simulink model "Modelo_NL_CONTROL_INTERNO_VECTORIAL"  (R2017a)
settings: Solver=VariableStepAuto  StartTime=0.0  StopTime=1  MaxStep=1e-4  RelTol=1e-3
values from neighbouring files (symbols this model uses):
  alfa_cu = 3.9e-3    (= 0.0039)    [modelo_global_NL.m]
  beq = bl/r^2 + bm    (= 1.5638971155e-05)    [Evaluacion_polos_5_2_2.m]    (also in modelo_global_NL.m = 1.5e-05)
  Cts = 0.818    [modelo_global_NL.m]
  Jeq = Jl/r^2 + Jm    (= 6.9338269301e-06)    [Evaluacion_polos_5_2_2.m]    (also in modelo_global_NL.m = 5.65588462007e-06)
  LambdaM = 0.01546    [Evaluacion_polos_5_2_2.m]    (also in modelo_global_NL.m)
  Ld = 0.0066    [Evaluacion_polos_5_2_2.m]    (also in modelo_global_NL.m)
  Lq = 0.0058    [Evaluacion_polos_5_2_2.m]    (also in modelo_global_NL.m)
  Pp = 3    [Evaluacion_polos_5_2_2.m]    (also in modelo_global_NL.m)
  R0 = 4    [Evaluacion_polos_5_2_2.m]    (also in modelo_global_NL.m)
  Rd = 33    [Evaluacion_polos_5_2_2.m]    (also in modelo_global_NL.m)
  Rq = 29    [Evaluacion_polos_5_2_2.m]    (also in modelo_global_NL.m)
  Rsref = 1.02    [modelo_global_NL.m]
  Rts_amb = 146.7    [modelo_global_NL.m]
  Tamb = 40    [modelo_global_NL.m]
  Tsref = 40    [modelo_global_NL.m]
undefined symbols (not defined in the file or in its folder): sigbuilder_block
settings Model: Creator=merem  LastModifiedBy=merem

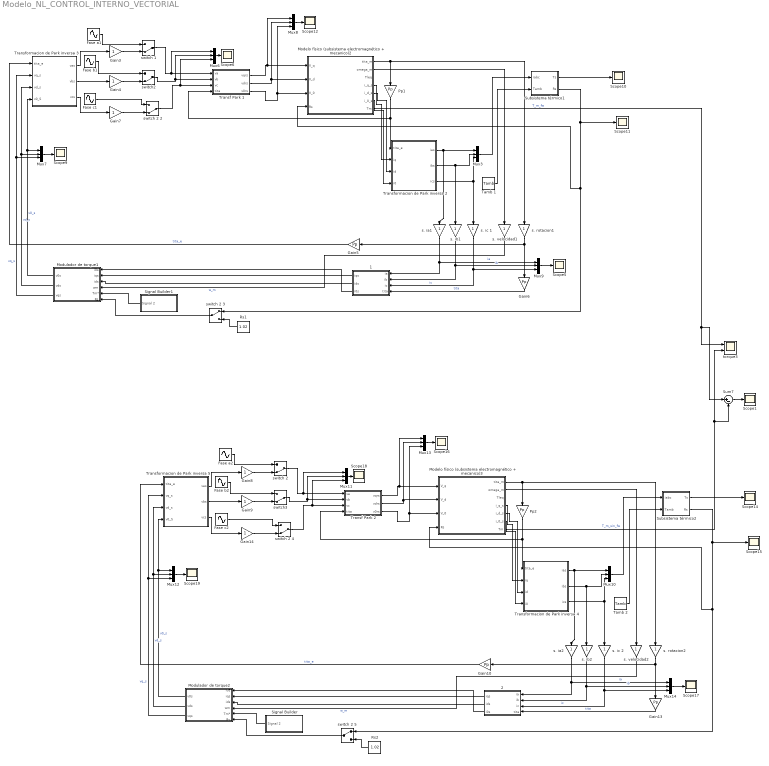
== system Modelo_NL_CONTROL_INTERNO_VECTORIAL ==
  " 1" : Subsystem
  " 2" : Subsystem
  Fase a1 : Sin  SampleTime=0
  Fase a2 : Sin  SampleTime=0
  Fase b1 : Sin  SampleTime=0
  Fase b2 : Sin  SampleTime=0
  Fase c1 : Sin  SampleTime=0
  Fase c2 : Sin  SampleTime=0
  Gain{5..6,10,13} (4 alike) : Gain  Gain=Pp
  Gain{3..4,7..9,14} (6 alike) : Gain
  Modelo físico (subsistema electromagnético + mecanico)2 : Subsystem
  Modelo físico (subsistema electromagnético + mecanico)3 : Subsystem
  Modulador de torque1 : Subsystem
  Modulador de torque2 : Subsystem
  Mux{3,6..14} (10 alike) : Mux  Inputs=3
  Pp1 : Gain  Gain=Pp
  Pp2 : Gain  Gain=Pp
  Rs1 : Constant  Value=1.02
  Rs2 : Constant  Value=1.02
  Scope{1,5..6,9..12,14..19} (13 alike) : Scope
  Signal Builder : Subsystem  Tag=STV Subsys  LoadFcn=sigbuilder_block('load');  StartFcn=sigbuilder_block('start');  StopFcn=sigbuilder_block('stop');  ClipboardFcn=sigbuilder_block('clipboard');  mask(Sigbuilder block){tuvar=[0:10]}
      mask help: Simulink:masks:SigbuilderBlock_MD
      mask init:
      | if ~strcmp(get_param(bdroot(gcbh),'SimulationStatus'),'stopped') tuvar = sigbuilder_block('maskInit'); end
      settings: CopyFcn=sigbuilder_block('copy');  DeleteFcn=sigbuilder_block('delete');  ModelCloseFcn=sigbuilder_block('modelClose');  PreSaveFcn=sigbuilder_block('preSave');  PauseFcn=sigbuilder_block('pause');  ContinueFcn=sigbuilder_block('continue');  NameChangeFcn=sigbuilder_block('namechange');  OpenFcn=sigbuilder_block('open',[6 30 1012.5 447.75 ]);  CloseFcn=sigbuilder_block('close');
      mask Display: plot(0, 0, 100, 100,[2, 2, 32, 32, 2], [68, 8, 8, 68, 68],[32, 2], [38, 38], [32, 19, 2],[53, 60, 44], [32, 17, 17, 2],[16, 16, 31, 31]);txt = getActiveGroup(gcbh);text(2, 100, txt,'verticalAlignment', 'top');
  Signal Builder1 : Subsystem  Tag=STV Subsys  LoadFcn=sigbuilder_block('load');  StartFcn=sigbuilder_block('start');  StopFcn=sigbuilder_block('stop');  ClipboardFcn=sigbuilder_block('clipboard');  mask(Sigbuilder block){tuvar=[0:10]}
      mask help: Simulink:masks:SigbuilderBlock_MD
      mask init:
      | if ~strcmp(get_param(bdroot(gcbh),'SimulationStatus'),'stopped') tuvar = sigbuilder_block('maskInit'); end
      settings: CopyFcn=sigbuilder_block('copy');  DeleteFcn=sigbuilder_block('delete');  ModelCloseFcn=sigbuilder_block('modelClose');  PreSaveFcn=sigbuilder_block('preSave');  PauseFcn=sigbuilder_block('pause');  ContinueFcn=sigbuilder_block('continue');  NameChangeFcn=sigbuilder_block('namechange');  OpenFcn=sigbuilder_block('open',[6 30 1012.5 447.75 ]);  CloseFcn=sigbuilder_block('close');
      mask Display: plot(0, 0, 100, 100,[2, 2, 32, 32, 2], [68, 8, 8, 68, 68],[32, 2], [38, 38], [32, 19, 2],[53, 60, 44], [32, 17, 17, 2],[16, 16, 31, 31]);txt = getActiveGroup(gcbh);text(2, 100, txt,'verticalAlignment', 'top');
  Subsistema térmico1 : Subsystem
  Subsistema térmico2 : Subsystem
  Sum7 : Sum  Inputs=|+-
  Tamb 1 : Constant  Value=Tamb
  Tamb 2 : Constant  Value=Tamb
  Transf Park 1 : Subsystem
  Transf Park 2 : Subsystem
  Transformacion de Park inversa 2 : Subsystem
  Transformacion de Park inversa 3 : Subsystem
  Transformacion de Park inversa 4 : Subsystem
  Transformacion de Park inversa 5 : Subsystem
  s. ia1 : Gain
  s. ia2 : Gain
  s. ib1 : Gain
  s. ib2 : Gain
  s. ic 1 : Gain
  s. ic 2 : Gain
  s. rotacion1 : Gain
  s. rotacion2 : Gain
  s. velocidad1 : Gain
  s. velocidad2 : Gain
  switch 1 : ManualSwitch  CurrentSetting=0
  switch 2 : ManualSwitch  CurrentSetting=0
  switch 2 2 : ManualSwitch  CurrentSetting=0
  switch 2 3 : ManualSwitch
  switch 2 4 : ManualSwitch  CurrentSetting=0
  switch 2 5 : ManualSwitch
  switch2 : ManualSwitch  CurrentSetting=0
  switch3 : ManualSwitch  CurrentSetting=0
  torque3 : Scope  NumInputPorts=2
  wires:
  Gain3/1 -> switch 1/2
  Modulador de torque1/2(vds) -> Mux7/2, Transformacion de Park inversa 3/3(vd_s)  "vd_s"
  " 1"/1(iqs) -> Modulador de torque1/2(iqs)
  Mux9/1 -> Scope5/1
  Gain6/1 -> " 1"/4("tita ")  "tita"
  s. rotacion1/1 -> Gain6/1, Gain5/1
  switch 2 2/1 -> Mux6/3, Transf Park 1/3(vc)
  Gain7/1 -> switch 2 2/2
  s. ib1/1 -> Mux9/2, " 1"/2("ib ")  "ib"
  Transformacion de Park inversa 2/3("ics ") -> Mux3/3, s. ic 1/1
  Gain4/1 -> switch2/2
  Fase c1/1 -> switch 2 2/1
  Subsistema térmico1/1(Ts) -> Scope10/1
  Transformacion de Park inversa 3/2(vbs) -> Gain4/1
  s. velocidad1/1 -> Modulador de torque1/4(wm)  "w_m"
  switch2/1 -> Mux6/2, Transf Park 1/2(vb)
  Modelo físico (subsistema electromagnético + mecanico)2/4("i_q_s ") -> Transformacion de Park inversa 2/2(iq)
  s. ia1/1 -> Mux9/1, " 1"/1("ia ")  "ia"
  Transf Park 1/2("vdrs ") -> Modelo físico (subsistema electromagnético + mecanico)2/2(V_d), Mux8/2
  Transformacion de Park inversa 2/1(ias) -> Mux3/1, s. ia1/1
  " 1"/2("ids ") -> Modulador de torque1/3(ids)
  Fase a1/1 -> switch 1/1
  s. ic 1/1 -> Mux9/3, " 1"/3("ic ")  "ic"
  switch 2 3/1 -> Modulador de torque1/6(Rs)
  Mux3/1 -> Subsistema térmico1/1(iabc)
  Transformacion de Park inversa 3/3("vcs ") -> Gain7/1
  Tamb 1/1 -> Subsistema térmico1/2("Tamb ")
  Modulador de torque1/3(vqs) -> Mux7/3, Transformacion de Park inversa 3/2(vq_s)  "vq_s"
  Mux7/1 -> Scope9/1
  Rs1/1 -> switch 2 3/2
  Pp1/1 -> Transf Park 1/4(tita), Transformacion de Park inversa 2/1(tita_e)
  " 1"/3("i0s ") -> Modulador de torque1/1(i0s)
  Transf Park 1/3("v0rs ") -> Modelo físico (subsistema electromagnético + mecanico)2/3(V_0), Mux8/3
  Transformacion de Park inversa 3/1(vas) -> Gain3/1
  Transf Park 1/1(vqrs) -> Modelo físico (subsistema electromagnético + mecanico)2/1(V_q), Mux8/1
  Fase b1/1 -> switch2/1
  switch 1/1 -> Mux6/1, Transf Park 1/1("va ")
  Mux8/1 -> Scope12/1
  Modelo físico (subsistema electromagnético + mecanico)2/6("i_0_s ") -> Transformacion de Park inversa 2/4(i0)
  Modelo físico (subsistema electromagnético + mecanico)2/5("i_d_s ") -> Transformacion de Park inversa 2/3(id)
  Transformacion de Park inversa 2/2(ibs) -> Mux3/2, s. ib1/1
  Modelo físico (subsistema electromagnético + mecanico)2/1("tita_m ") -> Pp1/1, s. rotacion1/1
  Subsistema térmico1/2("Rs ") -> Scope11/1, Modelo físico (subsistema electromagnético + mecanico)2/4(Rs), switch 2 3/1
  Modulador de torque1/1(v0s) -> Mux7/1, Transformacion de Park inversa 3/4("v0_S ")  "v0_s"
  Gain5/1 -> Transformacion de Park inversa 3/1(tita_e)  "tita_e"
  Mux6/1 -> Scope6/1
  Gain8/1 -> switch 2/2
  " 2"/1(iqs) -> Modulador de torque2/2(iqs)
  Modulador de torque2/2(vds) -> Mux12/2, Transformacion de Park inversa 5/3(vd_s)  "vd_s"
  Gain9/1 -> switch3/2
  s. velocidad2/1 -> Modulador de torque2/4(wm)  "w_m"
  Subsistema térmico2/1(Ts) -> Scope14/1
  s. ib2/1 -> Mux14/2, " 2"/2("ib ")  "ib"
  Gain14/1 -> switch 2 4/2
  Gain13/1 -> " 2"/4("tita ")  "tita"
  Transformacion de Park inversa 5/1(vas) -> Gain8/1
  Mux14/1 -> Scope17/1
  Gain10/1 -> Transformacion de Park inversa 5/1(tita_e)  "tita_e"
  Transformacion de Park inversa 4/2(ibs) -> Mux10/2, s. ib2/1
  Mux11/1 -> Scope18/1
  Modulador de torque2/1(v0s) -> Mux12/1, Transformacion de Park inversa 5/4("v0_S ")  "v0_s"
  Modelo físico (subsistema electromagnético + mecanico)3/5("i_d_s ") -> Transformacion de Park inversa 4/3(id)
  switch 2 4/1 -> Mux11/3, Transf Park 2/3(vc)
  Pp2/1 -> Transf Park 2/4(tita), Transformacion de Park inversa 4/1(tita_e)
  Transf Park 2/2("vdrs ") -> Modelo físico (subsistema electromagnético + mecanico)3/2(V_d), Mux13/2
  s. rotacion2/1 -> Gain13/1, Gain10/1
  Transformacion de Park inversa 5/3("vcs ") -> Gain14/1
  Modulador de torque2/3(vqs) -> Mux12/3, Transformacion de Park inversa 5/2(vq_s)  "vq_s"
  " 2"/2("ids ") -> Modulador de torque2/3(ids)
  Transformacion de Park inversa 5/2(vbs) -> Gain9/1
  s. ia2/1 -> Mux14/1, " 2"/1("ia ")  "ia"
  switch3/1 -> Mux11/2, Transf Park 2/2(vb)
  Modelo físico (subsistema electromagnético + mecanico)3/4("i_q_s ") -> Transformacion de Park inversa 4/2(iq)
  switch 2 5/1 -> Modulador de torque2/6(Rs)
  Fase c2/1 -> switch 2 4/1
  Modelo físico (subsistema electromagnético + mecanico)3/1("tita_m ") -> Pp2/1, s. rotacion2/1
  Transformacion de Park inversa 4/1(ias) -> Mux10/1, s. ia2/1
  Mux10/1 -> Subsistema térmico2/1(iabc)
  switch 2/1 -> Mux11/1, Transf Park 2/1("va ")
  Tamb 2/1 -> Subsistema térmico2/2("Tamb ")
  Transf Park 2/1(vqrs) -> Modelo físico (subsistema electromagnético + mecanico)3/1(V_q), Mux13/1
  Modelo físico (subsistema electromagnético + mecanico)3/6("i_0_s ") -> Transformacion de Park inversa 4/4(i0)
  Transformacion de Park inversa 4/3("ics ") -> Mux10/3, s. ic 2/1
  Mux12/1 -> Scope19/1
  " 2"/3("i0s ") -> Modulador de torque2/1(i0s)
  Mux13/1 -> Scope16/1
  Fase a2/1 -> switch 2/1
  s. ic 2/1 -> Mux14/3, " 2"/3("ic ")  "ic"
  Transf Park 2/3("v0rs ") -> Modelo físico (subsistema electromagnético + mecanico)3/3(V_0), Mux13/3
  Fase b2/1 -> switch3/1
  Rs2/1 -> switch 2 5/2
  Subsistema térmico2/2("Rs ") -> Scope15/1, Modelo físico (subsistema electromagnético + mecanico)3/4(Rs), switch 2 5/1
  Modelo físico (subsistema electromagnético + mecanico)3/7(Tm) -> Sum7/2, torque3/2  "T_m_sin_fw"
  Modelo físico (subsistema electromagnético + mecanico)2/7(Tm) -> Sum7/1, torque3/1  "T_m_fw"
  Signal Builder/1(Signal 2) -> Modulador de torque2/5(Tm*)
  Signal Builder1/1(Signal 2) -> Modulador de torque1/5(Tm*)
  Modelo físico (subsistema electromagnético + mecanico)2/2("omega_m ") -> s. velocidad1/1
  Modelo físico (subsistema electromagnético + mecanico)3/2("omega_m ") -> s. velocidad2/1
  Sum7/1 -> Scope1/1

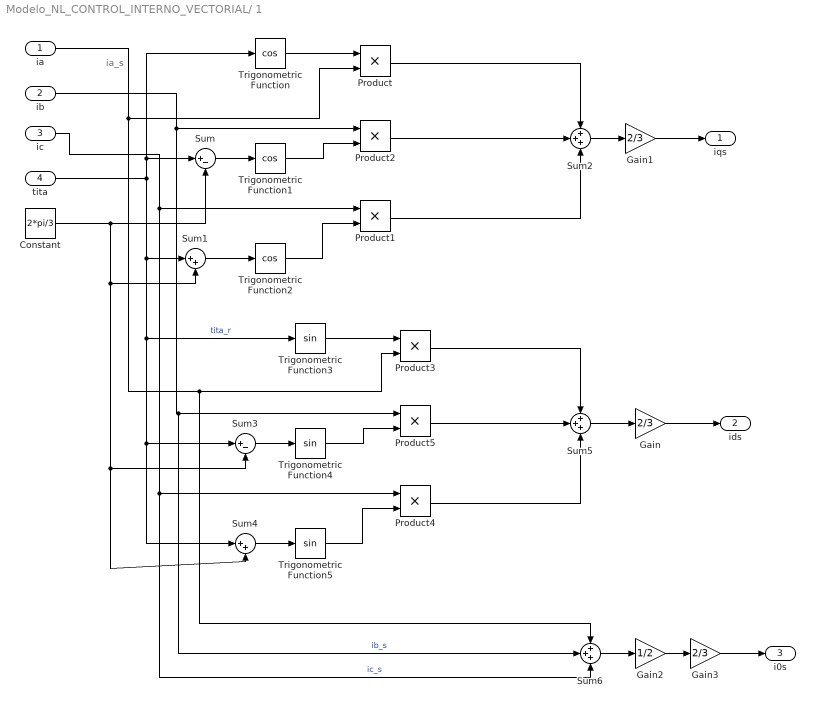
== system Modelo_NL_CONTROL_INTERNO_VECTORIAL/ 1 ==
  note: ia_s
  "ia " : Inport
  "ib " : Inport  Port=2
  "ic " : Inport  Port=3
  "tita " : Inport  Port=4
  Constant : Constant  Value=2*pi/3
  Gain : Gain  Gain=2/3
  Gain1 : Gain  Gain=2/3
  Gain2 : Gain  Gain=1/2
  Gain3 : Gain  Gain=2/3
  Product{,1..5} (6 alike) : Product
  Sum : Sum  Inputs=|+-
  Sum1 : Sum  Inputs=|++
  Sum2 : Sum  Inputs=+++
  Sum3 : Sum  Inputs=|+-
  Sum4 : Sum  Inputs=|++
  Sum5 : Sum  Inputs=+++
  Sum6 : Sum  Inputs=+++
  Trigonometric Function : Trigonometry  Operator=cos
  Trigonometric Function1 : Trigonometry  Operator=cos
  Trigonometric Function2 : Trigonometry  Operator=cos
  Trigonometric Function3 : Trigonometry
  Trigonometric Function4 : Trigonometry
  Trigonometric Function5 : Trigonometry
  iqs : Outport
  "ids " : Outport  Port=2
  "i0s " : Outport  Port=3
  wires:
  "tita "/1 -> Trigonometric Function/1, Sum/1, Sum1/1, Trigonometric Function3/1, Sum3/1, Sum4/1  "tita_r"
  Trigonometric Function/1 -> Product/1
  "ia "/1 -> Sum6/1, Product3/2, Product/2
  Constant/1 -> Sum4/2, Sum3/2, Sum1/2, Sum/2
  Sum/1 -> Trigonometric Function1/1
  Sum1/1 -> Trigonometric Function2/1
  Trigonometric Function1/1 -> Product2/2
  Trigonometric Function2/1 -> Product1/2
  "ib "/1 -> Sum6/2, Product5/1, Product2/1  "ib_s"
  "ic "/1 -> Sum6/3, Product4/1, Product1/1  "ic_s"
  Product/1 -> Sum2/1
  Product2/1 -> Sum2/2
  Sum2/1 -> Gain1/1
  Trigonometric Function5/1 -> Product4/2
  Trigonometric Function3/1 -> Product3/1
  Sum4/1 -> Trigonometric Function5/1
  Sum3/1 -> Trigonometric Function4/1
  Trigonometric Function4/1 -> Product5/2
  Product3/1 -> Sum5/1
  Product5/1 -> Sum5/2
  Product4/1 -> Sum5/3
  Sum5/1 -> Gain/1
  Product1/1 -> Sum2/3
  Gain/1 -> "ids "/1
  Gain1/1 -> iqs/1
  Sum6/1 -> Gain2/1
  Gain2/1 -> Gain3/1
  Gain3/1 -> "i0s "/1

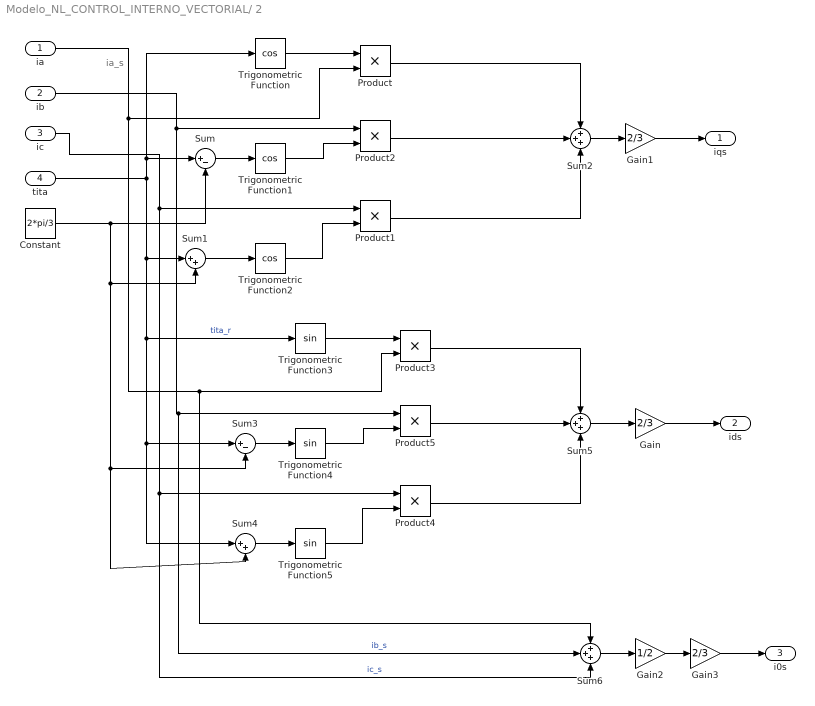
== system Modelo_NL_CONTROL_INTERNO_VECTORIAL/ 2 ==
  note: ia_s
  "ia " : Inport
  "ib " : Inport  Port=2
  "ic " : Inport  Port=3
  "tita " : Inport  Port=4
  Constant : Constant  Value=2*pi/3
  Gain : Gain  Gain=2/3
  Gain1 : Gain  Gain=2/3
  Gain2 : Gain  Gain=1/2
  Gain3 : Gain  Gain=2/3
  Product{,1..5} (6 alike) : Product
  Sum : Sum  Inputs=|+-
  Sum1 : Sum  Inputs=|++
  Sum2 : Sum  Inputs=+++
  Sum3 : Sum  Inputs=|+-
  Sum4 : Sum  Inputs=|++
  Sum5 : Sum  Inputs=+++
  Sum6 : Sum  Inputs=+++
  Trigonometric Function : Trigonometry  Operator=cos
  Trigonometric Function1 : Trigonometry  Operator=cos
  Trigonometric Function2 : Trigonometry  Operator=cos
  Trigonometric Function3 : Trigonometry
  Trigonometric Function4 : Trigonometry
  Trigonometric Function5 : Trigonometry
  iqs : Outport
  "ids " : Outport  Port=2
  "i0s " : Outport  Port=3
  wires:
  "tita "/1 -> Trigonometric Function/1, Sum/1, Sum1/1, Trigonometric Function3/1, Sum3/1, Sum4/1  "tita_r"
  Trigonometric Function/1 -> Product/1
  "ia "/1 -> Sum6/1, Product3/2, Product/2
  Constant/1 -> Sum4/2, Sum3/2, Sum1/2, Sum/2
  Sum/1 -> Trigonometric Function1/1
  Sum1/1 -> Trigonometric Function2/1
  Trigonometric Function1/1 -> Product2/2
  Trigonometric Function2/1 -> Product1/2
  "ib "/1 -> Sum6/2, Product5/1, Product2/1  "ib_s"
  "ic "/1 -> Sum6/3, Product4/1, Product1/1  "ic_s"
  Product/1 -> Sum2/1
  Product2/1 -> Sum2/2
  Sum2/1 -> Gain1/1
  Trigonometric Function5/1 -> Product4/2
  Trigonometric Function3/1 -> Product3/1
  Sum4/1 -> Trigonometric Function5/1
  Sum3/1 -> Trigonometric Function4/1
  Trigonometric Function4/1 -> Product5/2
  Product3/1 -> Sum5/1
  Product5/1 -> Sum5/2
  Product4/1 -> Sum5/3
  Sum5/1 -> Gain/1
  Product1/1 -> Sum2/3
  Gain/1 -> "ids "/1
  Gain1/1 -> iqs/1
  Sum6/1 -> Gain2/1
  Gain2/1 -> Gain3/1
  Gain3/1 -> "i0s "/1

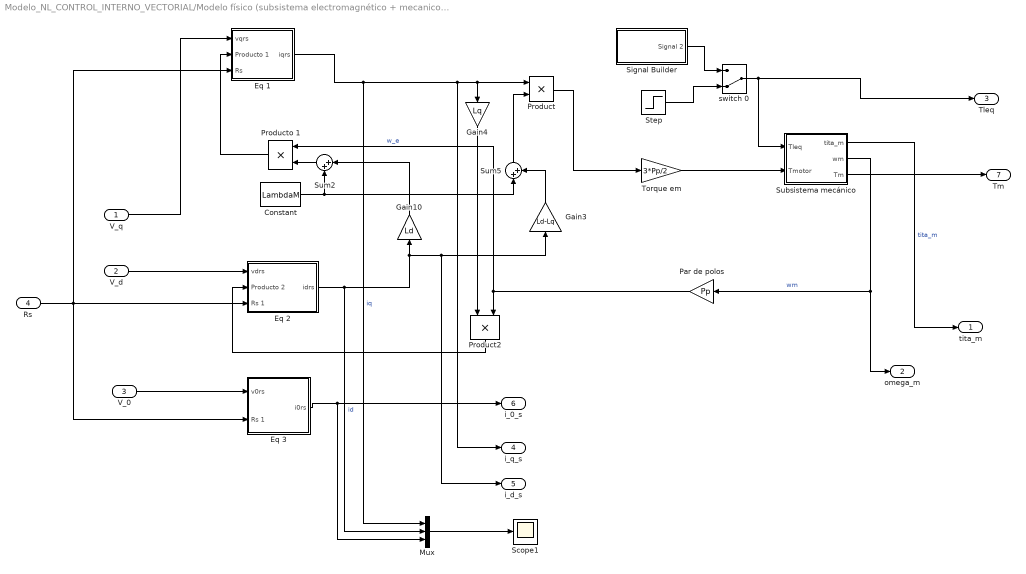
== system Modelo_NL_CONTROL_INTERNO_VECTORIAL/Modelo físico (subsistema electromagnético + mecanico)2 ==
  V_q : Inport
  V_d : Inport  Port=2
  V_0 : Inport  Port=3
  Rs : Inport  Port=4
  Constant : Constant  Value=LambdaM
  Eq 1 : Subsystem
  "Eq 2 " : Subsystem
  Eq 3 : Subsystem
  Gain10 : Gain  Gain=Ld
  Gain3 : Gain  Gain=Ld-Lq
  Gain4 : Gain  Gain=Lq
  Mux : Mux  Inputs=3
  Par de polos : Gain  Gain=Pp
  Product : Product
  Product2 : Product
  Producto 1 : Product
  Scope1 : Scope
  Signal Builder : Subsystem  Tag=STV Subsys  LoadFcn=sigbuilder_block('load');  StartFcn=sigbuilder_block('start');  StopFcn=sigbuilder_block('stop');  ClipboardFcn=sigbuilder_block('clipboard');  mask(Sigbuilder block){tuvar=[0:10]}
      mask help: Simulink:masks:SigbuilderBlock_MD
      mask init:
      | if ~strcmp(get_param(bdroot(gcbh),'SimulationStatus'),'stopped') tuvar = sigbuilder_block('maskInit'); end
      settings: CopyFcn=sigbuilder_block('copy');  DeleteFcn=sigbuilder_block('delete');  ModelCloseFcn=sigbuilder_block('modelClose');  PreSaveFcn=sigbuilder_block('preSave');  PauseFcn=sigbuilder_block('pause');  ContinueFcn=sigbuilder_block('continue');  NameChangeFcn=sigbuilder_block('namechange');  OpenFcn=sigbuilder_block('open',[6 30 1012.5 447.75 ]);  CloseFcn=sigbuilder_block('close');
      mask Display: plot(0, 0, 100, 100,[2, 2, 32, 32, 2], [68, 8, 8, 68, 68],[32, 2], [38, 38], [32, 19, 2],[53, 60, 44], [32, 17, 17, 2],[16, 16, 31, 31]);txt = getActiveGroup(gcbh);text(2, 100, txt,'verticalAlignment', 'top');
  Step : Step  Time=0.3  After=0  SampleTime=0
  Subsistema mecánico : Subsystem
  Sum2 : Sum  Inputs=|++
  Sum5 : Sum  Inputs=|++
  "Torque em " : Gain  Gain=3*Pp/2
  switch 0 : ManualSwitch  CurrentSetting=0
  "tita_m " : Outport
  "omega_m " : Outport  Port=2
  Tleq : Outport  Port=3
  "i_q_s " : Outport  Port=4
  "i_d_s " : Outport  Port=5
  "i_0_s " : Outport  Port=6
  Tm : Outport  Port=7
  wires:
  Sum2/1 -> Producto 1/2
  Sum5/1 -> Product/2
  Subsistema mecánico/2("wm ") -> "omega_m "/1, Par de polos/1  "wm"
  V_q/1 -> Eq 1/1(vqrs)
  Gain10/1 -> Sum2/1
  Par de polos/1 -> Producto 1/1, Product2/2  "w_e"
  "Torque em "/1 -> Subsistema mecánico/2("Tmotor ")
  Product/1 -> "Torque em "/1
  Constant/1 -> Sum5/1, Sum2/2
  Gain3/1 -> Sum5/2
  Gain4/1 -> Product2/1
  Eq 1/1("iqrs ") -> Mux/1, "i_q_s "/1, Gain4/1, Product/1  "iq"
  Subsistema mecánico/1("tita_m ") -> "tita_m "/1  "tita_m"
  "Eq 2 "/1("idrs ") -> Mux/2, "i_d_s "/1, Gain3/1, Gain10/1  "id"
  Product2/1 -> "Eq 2 "/2("Producto 2 ")
  Producto 1/1 -> Eq 1/2("Producto 1 ")
  V_d/1 -> "Eq 2 "/1("vdrs ")
  V_0/1 -> Eq 3/1("v0rs ")
  Eq 3/1("i0rs ") -> Mux/3, "i_0_s "/1
  Step/1 -> switch 0/2
  switch 0/1 -> Subsistema mecánico/1("Tleq "), Tleq/1
  Signal Builder/1(Signal 2) -> switch 0/1
  Rs/1 -> "Eq 2 "/3(Rs 1), Eq 3/2(Rs 1), Eq 1/3(Rs)
  Mux/1 -> Scope1/1
  Subsistema mecánico/3(Tm) -> Tm/1

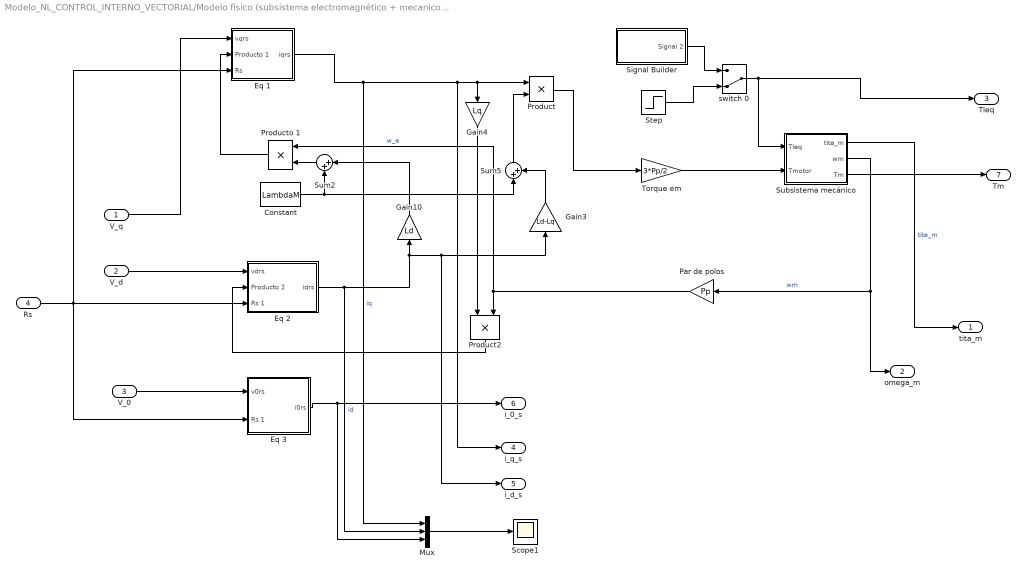
== system Modelo_NL_CONTROL_INTERNO_VECTORIAL/Modelo físico (subsistema electromagnético + mecanico)3 ==
  V_q : Inport
  V_d : Inport  Port=2
  V_0 : Inport  Port=3
  Rs : Inport  Port=4
  Constant : Constant  Value=LambdaM
  Eq 1 : Subsystem
  "Eq 2 " : Subsystem
  Eq 3 : Subsystem
  Gain10 : Gain  Gain=Ld
  Gain3 : Gain  Gain=Ld-Lq
  Gain4 : Gain  Gain=Lq
  Mux : Mux  Inputs=3
  Par de polos : Gain  Gain=Pp
  Product : Product
  Product2 : Product
  Producto 1 : Product
  Scope1 : Scope
  Signal Builder : Subsystem  Tag=STV Subsys  LoadFcn=sigbuilder_block('load');  StartFcn=sigbuilder_block('start');  StopFcn=sigbuilder_block('stop');  ClipboardFcn=sigbuilder_block('clipboard');  mask(Sigbuilder block){tuvar=[0:10]}
      mask help: Simulink:masks:SigbuilderBlock_MD
      mask init:
      | if ~strcmp(get_param(bdroot(gcbh),'SimulationStatus'),'stopped') tuvar = sigbuilder_block('maskInit'); end
      settings: CopyFcn=sigbuilder_block('copy');  DeleteFcn=sigbuilder_block('delete');  ModelCloseFcn=sigbuilder_block('modelClose');  PreSaveFcn=sigbuilder_block('preSave');  PauseFcn=sigbuilder_block('pause');  ContinueFcn=sigbuilder_block('continue');  NameChangeFcn=sigbuilder_block('namechange');  OpenFcn=sigbuilder_block('open',[6 30 1012.5 447.75 ]);  CloseFcn=sigbuilder_block('close');
      mask Display: plot(0, 0, 100, 100,[2, 2, 32, 32, 2], [68, 8, 8, 68, 68],[32, 2], [38, 38], [32, 19, 2],[53, 60, 44], [32, 17, 17, 2],[16, 16, 31, 31]);txt = getActiveGroup(gcbh);text(2, 100, txt,'verticalAlignment', 'top');
  Step : Step  Time=0.3  After=0  SampleTime=0
  Subsistema mecánico : Subsystem
  Sum2 : Sum  Inputs=|++
  Sum5 : Sum  Inputs=|++
  "Torque em " : Gain  Gain=3*Pp/2
  switch 0 : ManualSwitch  CurrentSetting=0
  "tita_m " : Outport
  "omega_m " : Outport  Port=2
  Tleq : Outport  Port=3
  "i_q_s " : Outport  Port=4
  "i_d_s " : Outport  Port=5
  "i_0_s " : Outport  Port=6
  Tm : Outport  Port=7
  wires:
  Sum2/1 -> Producto 1/2
  Sum5/1 -> Product/2
  Subsistema mecánico/2("wm ") -> "omega_m "/1, Par de polos/1  "wm"
  V_q/1 -> Eq 1/1(vqrs)
  Gain10/1 -> Sum2/1
  Par de polos/1 -> Producto 1/1, Product2/2  "w_e"
  "Torque em "/1 -> Subsistema mecánico/2("Tmotor ")
  Product/1 -> "Torque em "/1
  Constant/1 -> Sum5/1, Sum2/2
  Gain3/1 -> Sum5/2
  Gain4/1 -> Product2/1
  Eq 1/1("iqrs ") -> Mux/1, "i_q_s "/1, Gain4/1, Product/1  "iq"
  Subsistema mecánico/1("tita_m ") -> "tita_m "/1  "tita_m"
  "Eq 2 "/1("idrs ") -> Mux/2, "i_d_s "/1, Gain3/1, Gain10/1  "id"
  Product2/1 -> "Eq 2 "/2("Producto 2 ")
  Producto 1/1 -> Eq 1/2("Producto 1 ")
  V_d/1 -> "Eq 2 "/1("vdrs ")
  V_0/1 -> Eq 3/1("v0rs ")
  Eq 3/1("i0rs ") -> Mux/3, "i_0_s "/1
  Step/1 -> switch 0/2
  switch 0/1 -> Subsistema mecánico/1("Tleq "), Tleq/1
  Signal Builder/1(Signal 2) -> switch 0/1
  Rs/1 -> "Eq 2 "/3(Rs 1), Eq 3/2(Rs 1), Eq 1/3(Rs)
  Mux/1 -> Scope1/1
  Subsistema mecánico/3(Tm) -> Tm/1

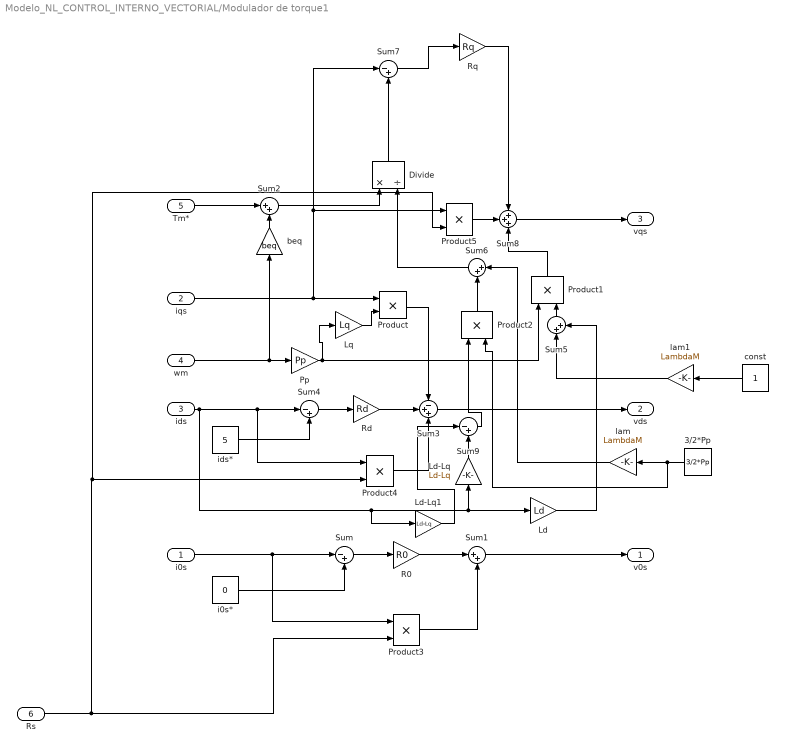
== system Modelo_NL_CONTROL_INTERNO_VECTORIAL/Modulador de torque1 ==
  i0s : Inport
  iqs : Inport  Port=2
  ids : Inport  Port=3
  wm : Inport  Port=4
  Tm* : Inport  Port=5
  Rs : Inport  Port=6
  3/2*Pp : Constant  Value=3/2*Pp
  Divide : Product  Inputs=*/
  Ld : Gain  Gain=Ld
  Ld-Lq : Gain  Gain=Ld-Lq
  Ld-Lq1 : Gain  Gain=Ld-Lq
  Lq : Gain  Gain=Lq
  Pp : Gain  Gain=Pp
  Product{,1..5} (6 alike) : Product
  R0 : Gain  Gain=R0
  Rd : Gain  Gain=Rd
  Rq : Gain  Gain=Rq
  Sum{,4,7,9} (4 alike) : Sum  Inputs=|-+
  Sum{1..2,5..6} (4 alike) : Sum  Inputs=|++
  Sum3 : Sum  Inputs=-++
  Sum8 : Sum  Inputs=+++
  beq : Gain  Gain=beq
  const : Constant
  i0s* : Constant  Value=0
  ids* : Constant  Value=5
  lam : Gain  Gain=LambdaM
  lam1 : Gain  Gain=LambdaM
  v0s : Outport
  vds : Outport  Port=2
  vqs : Outport  Port=3
  wires:
  i0s/1 -> Product3/1, Sum/1
  Sum1/1 -> v0s/1
  Product3/1 -> Sum1/2
  R0/1 -> Sum1/1
  Sum/1 -> R0/1
  i0s*/1 -> Sum/2
  Sum3/1 -> vds/1
  Sum4/1 -> Rd/1
  ids/1 -> Ld-Lq1/1, Ld/1, Ld-Lq/1, Product4/1, Sum4/1
  ids*/1 -> Sum4/2
  wm/1 -> Pp/1, beq/1
  Pp/1 -> Product1/1, Lq/1
  iqs/1 -> Product5/1, Sum7/1, Product/1
  Rd/1 -> Sum3/2
  Product/1 -> Sum3/1
  Tm*/1 -> Sum2/1
  beq/1 -> Sum2/2
  Sum5/1 -> Product1/2
  Ld/1 -> Sum5/2
  lam1/1 -> Sum5/1
  Sum2/1 -> Divide/1
  Sum7/1 -> Rq/1
  Rq/1 -> Sum8/1
  Product1/1 -> Sum8/3
  Sum8/1 -> vqs/1
  Product5/1 -> Sum8/2
  Product4/1 -> Sum3/3
  Lq/1 -> Product/2
  Sum6/1 -> Divide/2
  3/2*Pp/1 -> Product2/2, lam/1
  lam/1 -> Sum6/1
  Product2/1 -> Sum6/2
  const/1 -> lam1/1
  Rs/1 -> Product5/2, Product4/2, Product3/2
  Divide/1 -> Sum7/2
  Ld-Lq/1 -> Sum9/2
  Sum9/1 -> Product2/1
  Ld-Lq1/1 -> Sum9/1

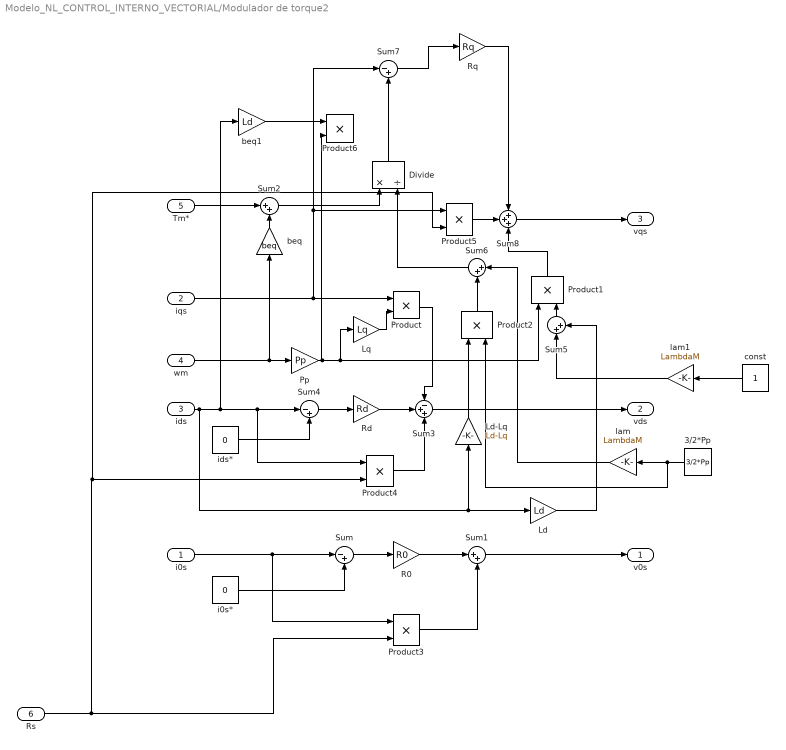
== system Modelo_NL_CONTROL_INTERNO_VECTORIAL/Modulador de torque2 ==
  i0s : Inport
  iqs : Inport  Port=2
  ids : Inport  Port=3
  wm : Inport  Port=4
  Tm* : Inport  Port=5
  Rs : Inport  Port=6
  3/2*Pp : Constant  Value=3/2*Pp
  Divide : Product  Inputs=*/
  Ld : Gain  Gain=Ld
  Ld-Lq : Gain  Gain=Ld-Lq
  Lq : Gain  Gain=Lq
  Pp : Gain  Gain=Pp
  Product{,1..6} (7 alike) : Product
  R0 : Gain  Gain=R0
  Rd : Gain  Gain=Rd
  Rq : Gain  Gain=Rq
  Sum : Sum  Inputs=|-+
  Sum{1..2,5..6} (4 alike) : Sum  Inputs=|++
  Sum3 : Sum  Inputs=-++
  Sum4 : Sum  Inputs=|-+
  Sum7 : Sum  Inputs=|-+
  Sum8 : Sum  Inputs=+++
  beq : Gain  Gain=beq
  beq1 : Gain  Gain=Ld
  const : Constant
  i0s* : Constant  Value=0
  ids* : Constant  Value=0
  lam : Gain  Gain=LambdaM
  lam1 : Gain  Gain=LambdaM
  v0s : Outport
  vds : Outport  Port=2
  vqs : Outport  Port=3
  wires:
  i0s/1 -> Product3/1, Sum/1
  Sum1/1 -> v0s/1
  Product3/1 -> Sum1/2
  R0/1 -> Sum1/1
  Sum/1 -> R0/1
  i0s*/1 -> Sum/2
  Sum3/1 -> vds/1
  Sum4/1 -> Rd/1
  ids/1 -> Ld/1, Ld-Lq/1, beq1/1, Product4/1, Sum4/1
  ids*/1 -> Sum4/2
  wm/1 -> Pp/1, beq/1
  Pp/1 -> Product1/1, Lq/1, Product6/2
  iqs/1 -> Product5/1, Sum7/1, Product/1
  Rd/1 -> Sum3/2
  Product/1 -> Sum3/1
  Tm*/1 -> Sum2/1
  beq/1 -> Sum2/2
  Sum5/1 -> Product1/2
  Ld/1 -> Sum5/2
  lam1/1 -> Sum5/1
  Sum2/1 -> Divide/1
  Sum7/1 -> Rq/1
  Rq/1 -> Sum8/1
  Product1/1 -> Sum8/3
  Sum8/1 -> vqs/1
  Product5/1 -> Sum8/2
  Product4/1 -> Sum3/3
  Lq/1 -> Product/2
  Sum6/1 -> Divide/2
  3/2*Pp/1 -> Product2/2, lam/1
  lam/1 -> Sum6/1
  Ld-Lq/1 -> Product2/1
  Product2/1 -> Sum6/2
  const/1 -> lam1/1
  Rs/1 -> Product5/2, Product4/2, Product3/2
  beq1/1 -> Product6/1
  Divide/1 -> Sum7/2

== system Modelo_NL_CONTROL_INTERNO_VECTORIAL/Signal Builder ==
  Demux : Demux  Tag=STV Demux  Outputs=1
  FromWs : FromWorkspace  Tag=STV FromWs  VariableName=tuvar  SampleTime=0
      SigBuilderData=|
      | common.afterFinalStr = 'Extrapolate'
      | common.sampleTime = 0
      | dataSet.timeRange = [0 2]
      | dataSet.name = 'Group 1'
      | sbobj.Groups.Name = 'Group 1'
      | sbobj.Groups.Signals.Name = 'Signal 2'
      | sbobj.Groups.Signals.XData = [0 0.3 0.3 0.5 0.5 0.9 0.9 2]
      | sbobj.Groups.Signals.YData = [0 0 0.025 0.025 -0.025 -0.025 0 0]
      | sbobj.Groups.TimeRange = [0 2]
  Signal 2 : Outport  Tag=STV Outport
  wires:
  FromWs/1 -> Demux/1
  Demux/1 -> Signal 2/1

== system Modelo_NL_CONTROL_INTERNO_VECTORIAL/Signal Builder1 ==
  Demux : Demux  Tag=STV Demux  Outputs=1
  FromWs : FromWorkspace  Tag=STV FromWs  VariableName=tuvar  SampleTime=0
      SigBuilderData=|
      | common.afterFinalStr = 'Extrapolate'
      | common.sampleTime = 0
      | dataSet.timeRange = [0 2]
      | dataSet.name = 'Group 1'
      | sbobj.Groups.Name = 'Group 1'
      | sbobj.Groups.Signals.Name = 'Signal 2'
      | sbobj.Groups.Signals.XData = [0 0.3 0.3 0.5 0.5 0.9 0.9 2]
      | sbobj.Groups.Signals.YData = [0 0 0.025 0.025 -0.025 -0.025 0 0]
      | sbobj.Groups.TimeRange = [0 2]
  Signal 2 : Outport  Tag=STV Outport
  wires:
  FromWs/1 -> Demux/1
  Demux/1 -> Signal 2/1

== system Modelo_NL_CONTROL_INTERNO_VECTORIAL/Subsistema térmico1 ==
  note: ib
  iabc : Inport
  "Tamb " : Inport  Port=2
  Constant : Constant  Value=Tsref
  Constant1 : Constant
  Demux : Demux  Outputs=3
  Gain : Gain  Gain=1/Cts
  Gain1 : Gain  Gain=1/Rts_amb
  Gain2 : Gain  Gain=alfa_cu
  Gain3 : Gain  Gain=Rsref
  Integrator : Integrator  InitialCondition=40
  Product{,1..3} (4 alike) : Product
  Sum : Sum  Inputs=+++
  Sum1 : Sum  Inputs=|+-
  Sum2 : Sum  Inputs=|+-
  Sum3 : Sum  Inputs=|++
  Sum4 : Sum  Inputs=|-+
  Ts : Outport
  "Rs " : Outport  Port=2
  wires:
  iabc/1 -> Demux/1
  Demux/1 -> Product/2, Product/1  "ia"
  Demux/2 -> Product1/2, Product1/1
  Demux/3 -> Product2/2, Product2/1  "ic"
  Product/1 -> Sum/1
  Product1/1 -> Sum/2
  Product2/1 -> Sum/3
  Sum/1 -> Product3/1
  Gain/1 -> Integrator/1
  Product3/1 -> Sum1/1
  Sum1/1 -> Gain/1
  Gain1/1 -> Sum1/2
  Integrator/1 -> Ts/1, Sum4/2, Sum2/1  "Ts"
  Constant/1 -> Sum2/2
  Sum2/1 -> Gain2/1
  Gain2/1 -> Sum3/1
  Constant1/1 -> Sum3/2
  Sum3/1 -> Gain3/1
  Gain3/1 -> "Rs "/1, Product3/2  "Rs"
  "Tamb "/1 -> Sum4/1
  Sum4/1 -> Gain1/1

== system Modelo_NL_CONTROL_INTERNO_VECTORIAL/Subsistema térmico2 ==
  note: ib
  iabc : Inport
  "Tamb " : Inport  Port=2
  Constant : Constant  Value=Tsref
  Constant1 : Constant
  Demux : Demux  Outputs=3
  Gain : Gain  Gain=1/Cts
  Gain1 : Gain  Gain=1/Rts_amb
  Gain2 : Gain  Gain=alfa_cu
  Gain3 : Gain  Gain=Rsref
  Integrator : Integrator  InitialCondition=40
  Product{,1..3} (4 alike) : Product
  Sum : Sum  Inputs=+++
  Sum1 : Sum  Inputs=|+-
  Sum2 : Sum  Inputs=|+-
  Sum3 : Sum  Inputs=|++
  Sum4 : Sum  Inputs=|-+
  Ts : Outport
  "Rs " : Outport  Port=2
  wires:
  iabc/1 -> Demux/1
  Demux/1 -> Product/2, Product/1  "ia"
  Demux/2 -> Product1/2, Product1/1
  Demux/3 -> Product2/2, Product2/1  "ic"
  Product/1 -> Sum/1
  Product1/1 -> Sum/2
  Product2/1 -> Sum/3
  Sum/1 -> Product3/1
  Gain/1 -> Integrator/1
  Product3/1 -> Sum1/1
  Sum1/1 -> Gain/1
  Gain1/1 -> Sum1/2
  Integrator/1 -> Ts/1, Sum4/2, Sum2/1  "Ts"
  Constant/1 -> Sum2/2
  Sum2/1 -> Gain2/1
  Gain2/1 -> Sum3/1
  Constant1/1 -> Sum3/2
  Sum3/1 -> Gain3/1
  Gain3/1 -> "Rs "/1, Product3/2  "Rs"
  "Tamb "/1 -> Sum4/1
  Sum4/1 -> Gain1/1

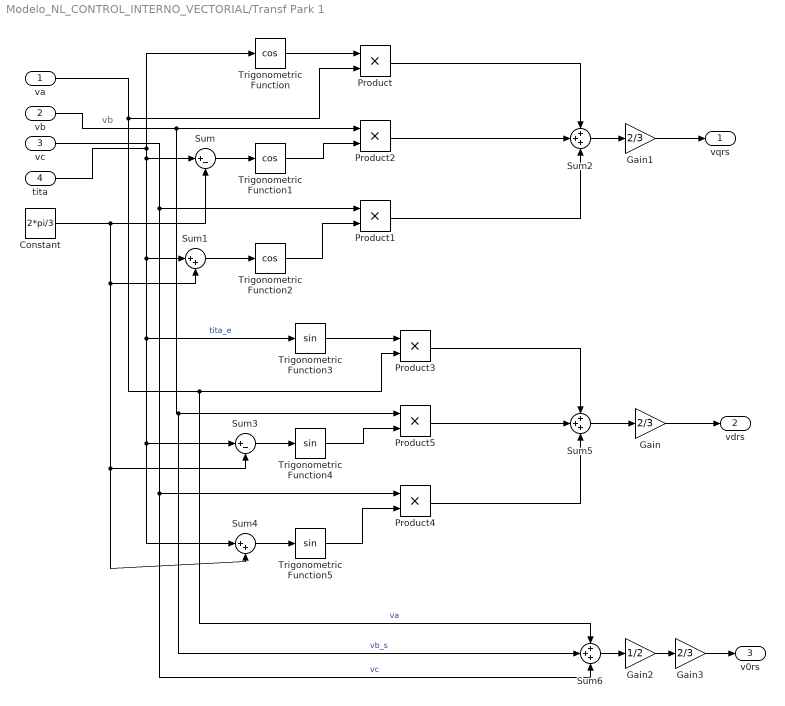
== system Modelo_NL_CONTROL_INTERNO_VECTORIAL/Transf Park 1 ==
  note: vb
  "va " : Inport
  vb : Inport  Port=2
  vc : Inport  Port=3
  tita : Inport  Port=4
  Constant : Constant  Value=2*pi/3
  Gain : Gain  Gain=2/3
  Gain1 : Gain  Gain=2/3
  Gain2 : Gain  Gain=1/2
  Gain3 : Gain  Gain=2/3
  Product{,1..5} (6 alike) : Product
  Sum : Sum  Inputs=|+-
  Sum1 : Sum  Inputs=|++
  Sum2 : Sum  Inputs=+++
  Sum3 : Sum  Inputs=|+-
  Sum4 : Sum  Inputs=|++
  Sum5 : Sum  Inputs=+++
  Sum6 : Sum  Inputs=+++
  Trigonometric Function : Trigonometry  Operator=cos
  Trigonometric Function1 : Trigonometry  Operator=cos
  Trigonometric Function2 : Trigonometry  Operator=cos
  Trigonometric Function3 : Trigonometry
  Trigonometric Function4 : Trigonometry
  Trigonometric Function5 : Trigonometry
  vqrs : Outport
  "vdrs " : Outport  Port=2
  "v0rs " : Outport  Port=3
  wires:
  tita/1 -> Sum1/1, Trigonometric Function3/1, Sum3/1, Sum4/1, Sum/1, Trigonometric Function/1  "tita_e"
  Trigonometric Function/1 -> Product/1
  "va "/1 -> Sum6/1, Product3/2, Product/2  "va"
  Constant/1 -> Sum4/2, Sum3/2, Sum1/2, Sum/2
  Sum/1 -> Trigonometric Function1/1
  Sum1/1 -> Trigonometric Function2/1
  Trigonometric Function1/1 -> Product2/2
  Trigonometric Function2/1 -> Product1/2
  vb/1 -> Sum6/2, Product5/1, Product2/1  "vb_s"
  vc/1 -> Sum6/3, Product4/1, Product1/1  "vc"
  Product/1 -> Sum2/1
  Product2/1 -> Sum2/2
  Sum2/1 -> Gain1/1
  Trigonometric Function5/1 -> Product4/2
  Trigonometric Function3/1 -> Product3/1
  Sum4/1 -> Trigonometric Function5/1
  Sum3/1 -> Trigonometric Function4/1
  Trigonometric Function4/1 -> Product5/2
  Product3/1 -> Sum5/1
  Product5/1 -> Sum5/2
  Product4/1 -> Sum5/3
  Sum5/1 -> Gain/1
  Product1/1 -> Sum2/3
  Gain/1 -> "vdrs "/1
  Gain1/1 -> vqrs/1
  Sum6/1 -> Gain2/1
  Gain3/1 -> "v0rs "/1
  Gain2/1 -> Gain3/1

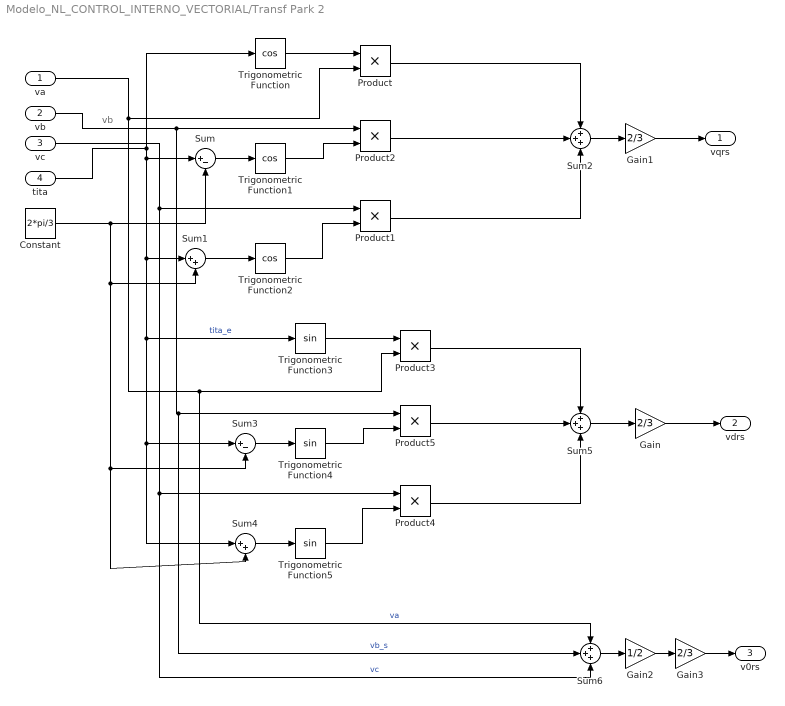
== system Modelo_NL_CONTROL_INTERNO_VECTORIAL/Transf Park 2 ==
  note: vb
  "va " : Inport
  vb : Inport  Port=2
  vc : Inport  Port=3
  tita : Inport  Port=4
  Constant : Constant  Value=2*pi/3
  Gain : Gain  Gain=2/3
  Gain1 : Gain  Gain=2/3
  Gain2 : Gain  Gain=1/2
  Gain3 : Gain  Gain=2/3
  Product{,1..5} (6 alike) : Product
  Sum : Sum  Inputs=|+-
  Sum1 : Sum  Inputs=|++
  Sum2 : Sum  Inputs=+++
  Sum3 : Sum  Inputs=|+-
  Sum4 : Sum  Inputs=|++
  Sum5 : Sum  Inputs=+++
  Sum6 : Sum  Inputs=+++
  Trigonometric Function : Trigonometry  Operator=cos
  Trigonometric Function1 : Trigonometry  Operator=cos
  Trigonometric Function2 : Trigonometry  Operator=cos
  Trigonometric Function3 : Trigonometry
  Trigonometric Function4 : Trigonometry
  Trigonometric Function5 : Trigonometry
  vqrs : Outport
  "vdrs " : Outport  Port=2
  "v0rs " : Outport  Port=3
  wires:
  tita/1 -> Sum1/1, Trigonometric Function3/1, Sum3/1, Sum4/1, Sum/1, Trigonometric Function/1  "tita_e"
  Trigonometric Function/1 -> Product/1
  "va "/1 -> Sum6/1, Product3/2, Product/2  "va"
  Constant/1 -> Sum4/2, Sum3/2, Sum1/2, Sum/2
  Sum/1 -> Trigonometric Function1/1
  Sum1/1 -> Trigonometric Function2/1
  Trigonometric Function1/1 -> Product2/2
  Trigonometric Function2/1 -> Product1/2
  vb/1 -> Sum6/2, Product5/1, Product2/1  "vb_s"
  vc/1 -> Sum6/3, Product4/1, Product1/1  "vc"
  Product/1 -> Sum2/1
  Product2/1 -> Sum2/2
  Sum2/1 -> Gain1/1
  Trigonometric Function5/1 -> Product4/2
  Trigonometric Function3/1 -> Product3/1
  Sum4/1 -> Trigonometric Function5/1
  Sum3/1 -> Trigonometric Function4/1
  Trigonometric Function4/1 -> Product5/2
  Product3/1 -> Sum5/1
  Product5/1 -> Sum5/2
  Product4/1 -> Sum5/3
  Sum5/1 -> Gain/1
  Product1/1 -> Sum2/3
  Gain/1 -> "vdrs "/1
  Gain1/1 -> vqrs/1
  Sum6/1 -> Gain2/1
  Gain3/1 -> "v0rs "/1
  Gain2/1 -> Gain3/1

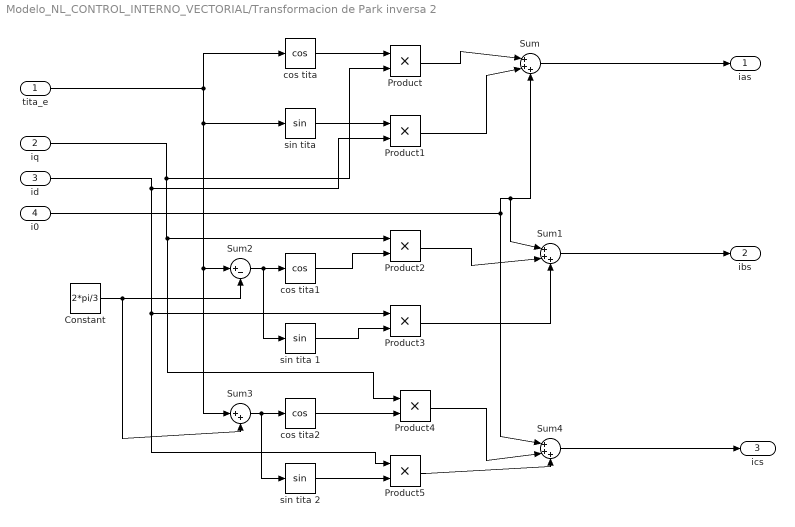
== system Modelo_NL_CONTROL_INTERNO_VECTORIAL/Transformacion de Park inversa 2 ==
  tita_e : Inport
  iq : Inport  Port=2
  id : Inport  Port=3
  i0 : Inport  Port=4
  Constant : Constant  Value=2*pi/3
  Product{,1..5} (6 alike) : Product
  Sum : Sum  Inputs=|+++
  Sum1 : Sum  Inputs=|+++
  Sum2 : Sum  Inputs=|+-
  Sum3 : Sum  Inputs=|++
  Sum4 : Sum  Inputs=|+++
  cos tita : Trigonometry  Operator=cos
  cos tita1 : Trigonometry  Operator=cos
  cos tita2 : Trigonometry  Operator=cos
  "sin tita " : Trigonometry
  sin tita 1 : Trigonometry
  sin tita 2 : Trigonometry
  ias : Outport
  ibs : Outport  Port=2
  "ics " : Outport  Port=3
  wires:
  tita_e/1 -> Sum3/1, Sum2/1, "sin tita "/1, cos tita/1
  iq/1 -> Product4/1, Product2/1, Product/2
  cos tita/1 -> Product/1
  "sin tita "/1 -> Product1/1
  id/1 -> Product5/1, Product3/1, Product1/2
  Product/1 -> Sum/1
  Product1/1 -> Sum/2
  Sum/1 -> ias/1
  i0/1 -> Sum1/1, Sum/3, Sum4/1
  cos tita1/1 -> Product2/2
  sin tita 1/1 -> Product3/2
  Product3/1 -> Sum1/3
  Product2/1 -> Sum1/2
  Sum1/1 -> ibs/1
  Constant/1 -> Sum3/2, Sum2/2
  Sum2/1 -> sin tita 1/1, cos tita1/1
  Sum3/1 -> sin tita 2/1, cos tita2/1
  cos tita2/1 -> Product4/2
  sin tita 2/1 -> Product5/2
  Product5/1 -> Sum4/3
  Product4/1 -> Sum4/2
  Sum4/1 -> "ics "/1

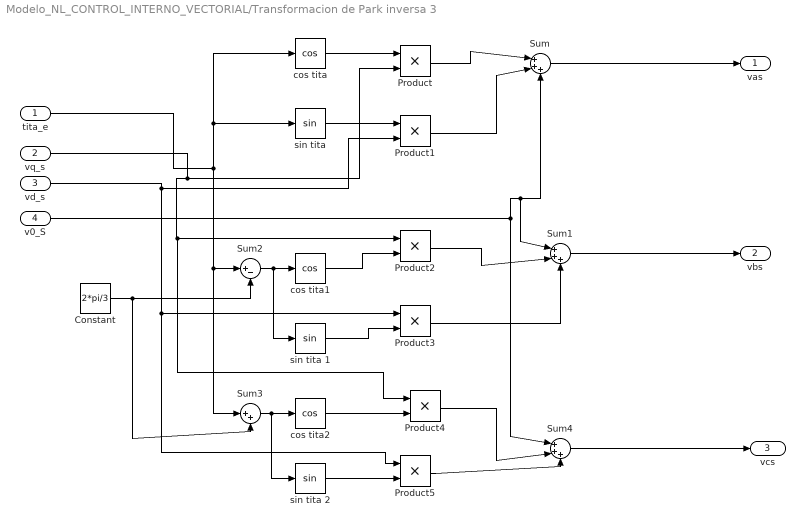
== system Modelo_NL_CONTROL_INTERNO_VECTORIAL/Transformacion de Park inversa 3 ==
  tita_e : Inport
  vq_s : Inport  Port=2
  vd_s : Inport  Port=3
  "v0_S " : Inport  Port=4
  Constant : Constant  Value=2*pi/3
  Product{,1..5} (6 alike) : Product
  Sum : Sum  Inputs=|+++
  Sum1 : Sum  Inputs=|+++
  Sum2 : Sum  Inputs=|+-
  Sum3 : Sum  Inputs=|++
  Sum4 : Sum  Inputs=|+++
  cos tita : Trigonometry  Operator=cos
  cos tita1 : Trigonometry  Operator=cos
  cos tita2 : Trigonometry  Operator=cos
  "sin tita " : Trigonometry
  sin tita 1 : Trigonometry
  sin tita 2 : Trigonometry
  vas : Outport
  vbs : Outport  Port=2
  "vcs " : Outport  Port=3
  wires:
  tita_e/1 -> Sum3/1, Sum2/1, cos tita/1, "sin tita "/1
  vq_s/1 -> Product4/1, Product2/1, Product/2
  cos tita/1 -> Product/1
  "sin tita "/1 -> Product1/1
  vd_s/1 -> Product5/1, Product3/1, Product1/2
  Product/1 -> Sum/1
  Product1/1 -> Sum/2
  Sum/1 -> vas/1
  "v0_S "/1 -> Sum1/1, Sum/3, Sum4/1
  cos tita1/1 -> Product2/2
  sin tita 1/1 -> Product3/2
  Product3/1 -> Sum1/3
  Product2/1 -> Sum1/2
  Sum1/1 -> vbs/1
  Constant/1 -> Sum3/2, Sum2/2
  Sum2/1 -> sin tita 1/1, cos tita1/1
  Sum3/1 -> sin tita 2/1, cos tita2/1
  cos tita2/1 -> Product4/2
  sin tita 2/1 -> Product5/2
  Product5/1 -> Sum4/3
  Product4/1 -> Sum4/2
  Sum4/1 -> "vcs "/1

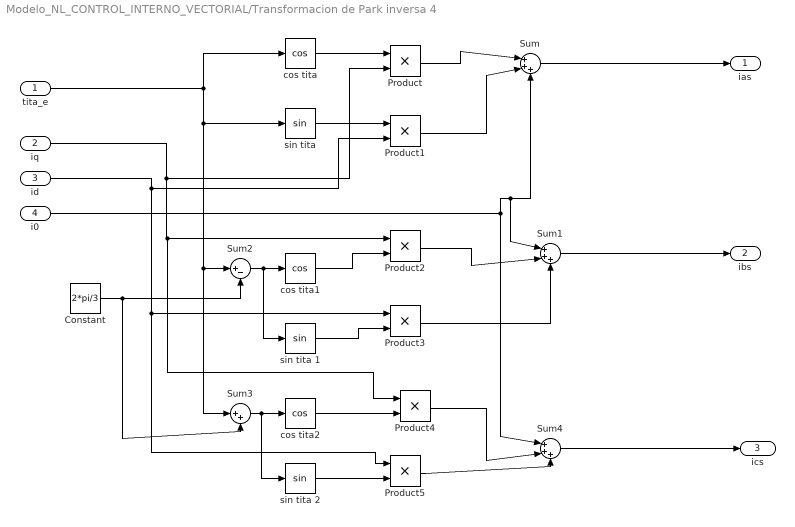
== system Modelo_NL_CONTROL_INTERNO_VECTORIAL/Transformacion de Park inversa 4 ==
  tita_e : Inport
  iq : Inport  Port=2
  id : Inport  Port=3
  i0 : Inport  Port=4
  Constant : Constant  Value=2*pi/3
  Product{,1..5} (6 alike) : Product
  Sum : Sum  Inputs=|+++
  Sum1 : Sum  Inputs=|+++
  Sum2 : Sum  Inputs=|+-
  Sum3 : Sum  Inputs=|++
  Sum4 : Sum  Inputs=|+++
  cos tita : Trigonometry  Operator=cos
  cos tita1 : Trigonometry  Operator=cos
  cos tita2 : Trigonometry  Operator=cos
  "sin tita " : Trigonometry
  sin tita 1 : Trigonometry
  sin tita 2 : Trigonometry
  ias : Outport
  ibs : Outport  Port=2
  "ics " : Outport  Port=3
  wires:
  tita_e/1 -> Sum3/1, Sum2/1, "sin tita "/1, cos tita/1
  iq/1 -> Product4/1, Product2/1, Product/2
  cos tita/1 -> Product/1
  "sin tita "/1 -> Product1/1
  id/1 -> Product5/1, Product3/1, Product1/2
  Product/1 -> Sum/1
  Product1/1 -> Sum/2
  Sum/1 -> ias/1
  i0/1 -> Sum1/1, Sum/3, Sum4/1
  cos tita1/1 -> Product2/2
  sin tita 1/1 -> Product3/2
  Product3/1 -> Sum1/3
  Product2/1 -> Sum1/2
  Sum1/1 -> ibs/1
  Constant/1 -> Sum3/2, Sum2/2
  Sum2/1 -> sin tita 1/1, cos tita1/1
  Sum3/1 -> sin tita 2/1, cos tita2/1
  cos tita2/1 -> Product4/2
  sin tita 2/1 -> Product5/2
  Product5/1 -> Sum4/3
  Product4/1 -> Sum4/2
  Sum4/1 -> "ics "/1

== system Modelo_NL_CONTROL_INTERNO_VECTORIAL/Transformacion de Park inversa 5 ==
  tita_e : Inport
  vq_s : Inport  Port=2
  vd_s : Inport  Port=3
  "v0_S " : Inport  Port=4
  Constant : Constant  Value=2*pi/3
  Product{,1..5} (6 alike) : Product
  Sum : Sum  Inputs=|+++
  Sum1 : Sum  Inputs=|+++
  Sum2 : Sum  Inputs=|+-
  Sum3 : Sum  Inputs=|++
  Sum4 : Sum  Inputs=|+++
  cos tita : Trigonometry  Operator=cos
  cos tita1 : Trigonometry  Operator=cos
  cos tita2 : Trigonometry  Operator=cos
  "sin tita " : Trigonometry
  sin tita 1 : Trigonometry
  sin tita 2 : Trigonometry
  vas : Outport
  vbs : Outport  Port=2
  "vcs " : Outport  Port=3
  wires:
  tita_e/1 -> Sum3/1, Sum2/1, cos tita/1, "sin tita "/1
  vq_s/1 -> Product4/1, Product2/1, Product/2
  cos tita/1 -> Product/1
  "sin tita "/1 -> Product1/1
  vd_s/1 -> Product5/1, Product3/1, Product1/2
  Product/1 -> Sum/1
  Product1/1 -> Sum/2
  Sum/1 -> vas/1
  "v0_S "/1 -> Sum1/1, Sum/3, Sum4/1
  cos tita1/1 -> Product2/2
  sin tita 1/1 -> Product3/2
  Product3/1 -> Sum1/3
  Product2/1 -> Sum1/2
  Sum1/1 -> vbs/1
  Constant/1 -> Sum3/2, Sum2/2
  Sum2/1 -> sin tita 1/1, cos tita1/1
  Sum3/1 -> sin tita 2/1, cos tita2/1
  cos tita2/1 -> Product4/2
  sin tita 2/1 -> Product5/2
  Product5/1 -> Sum4/3
  Product4/1 -> Sum4/2
  Sum4/1 -> "vcs "/1

== system Modelo_NL_CONTROL_INTERNO_VECTORIAL/Modelo físico (subsistema electromagnético + mecanico)2/Eq 1 ==
  vqrs : Inport
  "Producto 1 " : Inport  Port=2
  Rs : Inport  Port=3
  Gain : Gain  Gain=1/Lq
  Integrator : Integrator
  Product : Product
  Sum : Sum  Inputs=+--
  "iqrs " : Outport
  wires:
  Gain/1 -> Integrator/1
  Sum/1 -> Gain/1
  vqrs/1 -> Sum/1
  Product/1 -> Sum/2
  "Producto 1 "/1 -> Sum/3
  Integrator/1 -> Product/1, "iqrs "/1  "i_qs"
  Rs/1 -> Product/2

== system Modelo_NL_CONTROL_INTERNO_VECTORIAL/Modelo físico (subsistema electromagnético + mecanico)2/Eq 2  ==
  "vdrs " : Inport
  "Producto 2 " : Inport  Port=2
  Rs 1 : Inport  Port=3
  Gain2 : Gain  Gain=1/Ld
  Integrator1 : Integrator
  Product : Product
  Sum1 : Sum  Inputs=|+-+
  "idrs " : Outport
  wires:
  "Producto 2 "/1 -> Sum1/3
  Gain2/1 -> Integrator1/1
  Product/1 -> Sum1/2
  Sum1/1 -> Gain2/1
  Integrator1/1 -> Product/1, "idrs "/1  "i_ds"
  "vdrs "/1 -> Sum1/1
  Rs 1/1 -> Product/2

== system Modelo_NL_CONTROL_INTERNO_VECTORIAL/Modelo físico (subsistema electromagnético + mecanico)2/Eq 3 ==
  "v0rs " : Inport
  Rs 1 : Inport  Port=2
  Gain12 : Gain
  Integrator5 : Integrator
  Producto 1 : Product
  Sum4 : Sum  Inputs=|++
  "i0rs " : Outport
  wires:
  Gain12/1 -> Integrator5/1
  Sum4/1 -> Gain12/1
  Producto 1/1 -> Sum4/2
  "v0rs "/1 -> Sum4/1
  Integrator5/1 -> Producto 1/1, "i0rs "/1  "i_0s"

== system Modelo_NL_CONTROL_INTERNO_VECTORIAL/Modelo físico (subsistema electromagnético + mecanico)2/Signal Builder ==
  Demux : Demux  Tag=STV Demux  Outputs=1
  FromWs : FromWorkspace  Tag=STV FromWs  VariableName=tuvar  SampleTime=0
      SigBuilderData=|
      | common.afterFinalStr = 'Extrapolate'
      | common.sampleTime = 0
      | dataSet.timeRange = [0 2]
      | dataSet.name = 'Group 1'
      | sbobj.Groups.Name = 'Group 1'
      | sbobj.Groups.Signals.Name = 'Signal 2'
      | sbobj.Groups.Signals.XData = [0 0.3 0.3 0.5 0.5 0.9 0.9 2]
      | sbobj.Groups.Signals.YData = [0 0 0.02 0.02 -0.02 -0.02 0 0]
      | sbobj.Groups.TimeRange = [0 2]
  Signal 2 : Outport  Tag=STV Outport
  wires:
  FromWs/1 -> Demux/1
  Demux/1 -> Signal 2/1

== system Modelo_NL_CONTROL_INTERNO_VECTORIAL/Modelo físico (subsistema electromagnético + mecanico)2/Subsistema mecánico ==
  "Tleq " : Inport
  "Tmotor " : Inport  Port=2
  Gain6 : Gain  Gain=1/Jeq
  Gain8 : Gain  Gain=beq
  Integrator3 : Integrator
  Integrator4 : Integrator
  Sum3 : Sum  Inputs=-+-
  "tita_m " : Outport
  "wm " : Outport  Port=2
  Tm : Outport  Port=3
  wires:
  Integrator3/1 -> "tita_m "/1
  Integrator4/1 -> Gain8/1, "wm "/1, Integrator3/1
  Sum3/1 -> Tm/1, Gain6/1
  Gain6/1 -> Integrator4/1
  Gain8/1 -> Sum3/3
  "Tleq "/1 -> Sum3/1
  "Tmotor "/1 -> Sum3/2

== system Modelo_NL_CONTROL_INTERNO_VECTORIAL/Modelo físico (subsistema electromagnético + mecanico)3/Eq 1 ==
  vqrs : Inport
  "Producto 1 " : Inport  Port=2
  Rs : Inport  Port=3
  Gain : Gain  Gain=1/Lq
  Integrator : Integrator
  Product : Product
  Sum : Sum  Inputs=+--
  "iqrs " : Outport
  wires:
  Gain/1 -> Integrator/1
  Sum/1 -> Gain/1
  vqrs/1 -> Sum/1
  Product/1 -> Sum/2
  "Producto 1 "/1 -> Sum/3
  Integrator/1 -> Product/1, "iqrs "/1  "i_qs"
  Rs/1 -> Product/2

== system Modelo_NL_CONTROL_INTERNO_VECTORIAL/Modelo físico (subsistema electromagnético + mecanico)3/Eq 2  ==
  "vdrs " : Inport
  "Producto 2 " : Inport  Port=2
  Rs 1 : Inport  Port=3
  Gain2 : Gain  Gain=1/Ld
  Integrator1 : Integrator
  Product : Product
  Sum1 : Sum  Inputs=|+-+
  "idrs " : Outport
  wires:
  "Producto 2 "/1 -> Sum1/3
  Gain2/1 -> Integrator1/1
  Product/1 -> Sum1/2
  Sum1/1 -> Gain2/1
  Integrator1/1 -> Product/1, "idrs "/1  "i_ds"
  "vdrs "/1 -> Sum1/1
  Rs 1/1 -> Product/2

== system Modelo_NL_CONTROL_INTERNO_VECTORIAL/Modelo físico (subsistema electromagnético + mecanico)3/Eq 3 ==
  "v0rs " : Inport
  Rs 1 : Inport  Port=2
  Gain12 : Gain
  Integrator5 : Integrator
  Producto 1 : Product
  Sum4 : Sum  Inputs=|++
  "i0rs " : Outport
  wires:
  Gain12/1 -> Integrator5/1
  Sum4/1 -> Gain12/1
  Producto 1/1 -> Sum4/2
  "v0rs "/1 -> Sum4/1
  Integrator5/1 -> Producto 1/1, "i0rs "/1  "i_0s"

== system Modelo_NL_CONTROL_INTERNO_VECTORIAL/Modelo físico (subsistema electromagnético + mecanico)3/Signal Builder ==
  Demux : Demux  Tag=STV Demux  Outputs=1
  FromWs : FromWorkspace  Tag=STV FromWs  VariableName=tuvar  SampleTime=0
      SigBuilderData=|
      | common.afterFinalStr = 'Extrapolate'
      | common.sampleTime = 0
      | dataSet.timeRange = [0 2]
      | dataSet.name = 'Group 1'
      | sbobj.Groups.Name = 'Group 1'
      | sbobj.Groups.Signals.Name = 'Signal 2'
      | sbobj.Groups.Signals.XData = [0 0.3 0.3 0.5 0.5 0.9 0.9 2]
      | sbobj.Groups.Signals.YData = [0 0 0.02 0.02 -0.02 -0.02 0 0]
      | sbobj.Groups.TimeRange = [0 2]
  Signal 2 : Outport  Tag=STV Outport
  wires:
  FromWs/1 -> Demux/1
  Demux/1 -> Signal 2/1

== system Modelo_NL_CONTROL_INTERNO_VECTORIAL/Modelo físico (subsistema electromagnético + mecanico)3/Subsistema mecánico ==
  "Tleq " : Inport
  "Tmotor " : Inport  Port=2
  Gain6 : Gain  Gain=1/Jeq
  Gain8 : Gain  Gain=beq
  Integrator3 : Integrator
  Integrator4 : Integrator
  Scope15 : Scope
  Sum3 : Sum  Inputs=-+-
  "tita_m " : Outport
  "wm " : Outport  Port=2
  Tm : Outport  Port=3
  wires:
  Integrator3/1 -> "tita_m "/1
  Integrator4/1 -> Gain8/1, "wm "/1, Integrator3/1
  Sum3/1 -> Scope15/1, Tm/1, Gain6/1
  Gain6/1 -> Integrator4/1
  Gain8/1 -> Sum3/3
  "Tleq "/1 -> Sum3/1
  "Tmotor "/1 -> Sum3/2
